simulink model "PID_SpeedController"  (R2025a)
settings: Solver=FixedStepDiscrete  StartTime=0.0  StopTime=100  FixedStep=0.01  RelTol=1e-3
undefined symbols (not defined in the file or in its folder): DiscIntNeverNeededParam
libraries: simulink x1
settings Model: Creator=wangtianqi  LastModifiedBy=wangtianqi

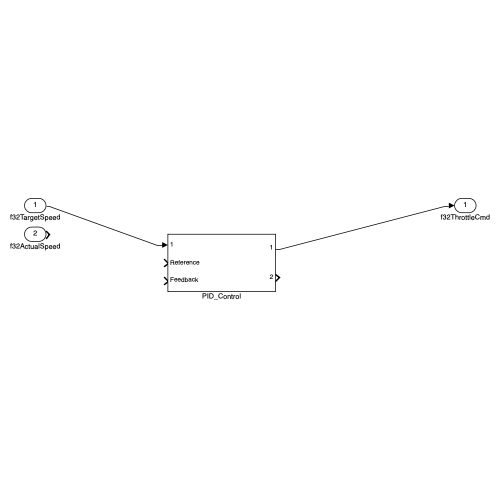
[thumbnail: Simulink's stored preview of the top-level diagram]
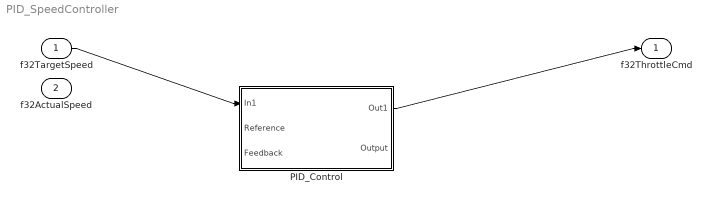
== system PID_SpeedController ==
  f32TargetSpeed : Inport  OutDataTypeStr=single
  f32ActualSpeed : Inport  Port=2  OutDataTypeStr=single
  PID_Control : Subsystem
  f32ThrottleCmd : Outport  OutDataTypeStr=single
  wires:
  f32TargetSpeed/1 -> PID_Control/1(In1)
  PID_Control/1(Out1) -> f32ThrottleCmd/1

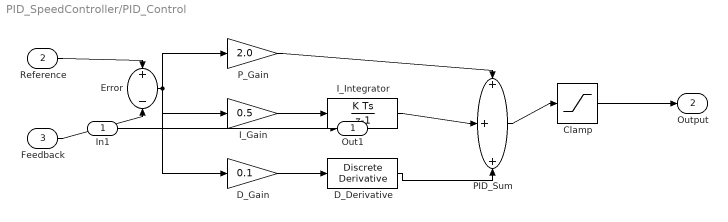
== system PID_SpeedController/PID_Control ==
  In1 : Inport
  Reference : Inport  Port=2
  Feedback : Inport  Port=3
  Clamp : Saturate  OutDataTypeStr=single
  D_Derivative : simulink/Discrete/Discrete Derivative  gainval=1.0  ICPrevScaledInput=0.0  OutMin=[]  OutMax=[]  OutDataTypeStr=single  OutputDataTypeScalingMode=single  OutDataType=fixdt(1, 16)  OutScaling=2^-10  DoSatur=off
  D_Gain : Gain  Gain=0.1  OutDataTypeStr=single
  Error : Sum  Inputs=+-  OutDataTypeStr=single
  I_Gain : Gain  Gain=0.5  OutDataTypeStr=single
  I_Integrator : DiscreteIntegrator  SampleTime=-1  OutDataTypeStr=single  ICPrevOutput=DiscIntNeverNeededParam  ICPrevScaledInput=DiscIntNeverNeededParam
  PID_Sum : Sum  Inputs=+++  OutDataTypeStr=single
  P_Gain : Gain  Gain=2.0  OutDataTypeStr=single
  Out1 : Outport
  Output : Outport  Port=2
  wires:
  In1/1 -> Out1/1
  Reference/1 -> Error/1
  Feedback/1 -> Error/2
  Error/1 -> P_Gain/1, I_Gain/1, D_Gain/1
  P_Gain/1 -> PID_Sum/1
  I_Gain/1 -> I_Integrator/1
  I_Integrator/1 -> PID_Sum/2
  D_Gain/1 -> D_Derivative/1
  D_Derivative/1 -> PID_Sum/3
  PID_Sum/1 -> Clamp/1
  Clamp/1 -> Output/1
